simulink model "SimulinkModel"  (R2013a)
settings: Solver=ode45  StartTime=0.0  StopTime=10.0  RelTol=1e-3
settings Model: Creator=andre  LastModifiedBy=andre

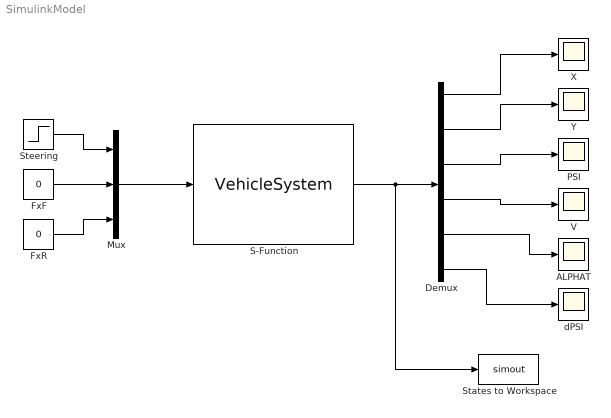
== system SimulinkModel ==
  ALPHAT : Scope
      settings: SaveName=ScopeData4
  Demux : Demux  Outputs=6
  FxF : Constant  Value=0
  FxR : Constant  Value=0
  Mux : Mux  Inputs=3
  PSI : Scope
      settings: SaveName=ScopeData2
  S-Function : S-Function  FunctionName=VehicleSystem  EnableBusSupport=off
  States to Workspace : ToWorkspace  VariableName=simout  SampleTime=-1  SaveFormat=Timeseries
  Steering : Step  After=5*pi/180  SampleTime=0
  V : Scope
      settings: SaveName=ScopeData3
  X : Scope
  Y : Scope
  dPSI : Scope
      settings: SaveName=ScopeData5
  wires:
  Steering/1 -> Mux/1
  FxF/1 -> Mux/2
  FxR/1 -> Mux/3
  Mux/1 -> S-Function/1
  S-Function/1 -> States to Workspace/1, Demux/1
  Demux/1 -> X/1
  Demux/2 -> Y/1
  Demux/3 -> PSI/1
  Demux/4 -> V/1
  Demux/5 -> ALPHAT/1
  Demux/6 -> dPSI/1
